simulink model "delay_tuning"  (R2019a)
settings: Solver=VariableStepAuto  StartTime=0.0  StopTime=.05  RelTol=1e-3
values from neighbouring files (symbols this model uses):
  Ari = double(Ari)    [StateSpaceController.m]
  Bri = double(Bri)    [StateSpaceController.m]
  Cri = eye(size(Ari,1))    [StateSpaceController.m]
  Dri = zeros(size(Bri))    [StateSpaceController.m]
  Krv = lqr(Ari, Bri, Qv, diag([0.3 0.3 0.47]) )    [StateSpaceController.m]
  roll_control_delay = ss(Ari, Bri, Cri, Dri, 'InputDelay',[0.07 0.07 0.01])    [StateSpaceController.m]
undefined symbols (not defined in the file or in its folder): e0_0, e1_0, e2_0, e3_0, masscgI
libraries: sharedtransform x3, sharedutil x1
settings Model: Creator=rag  LastModifiedBy=rag

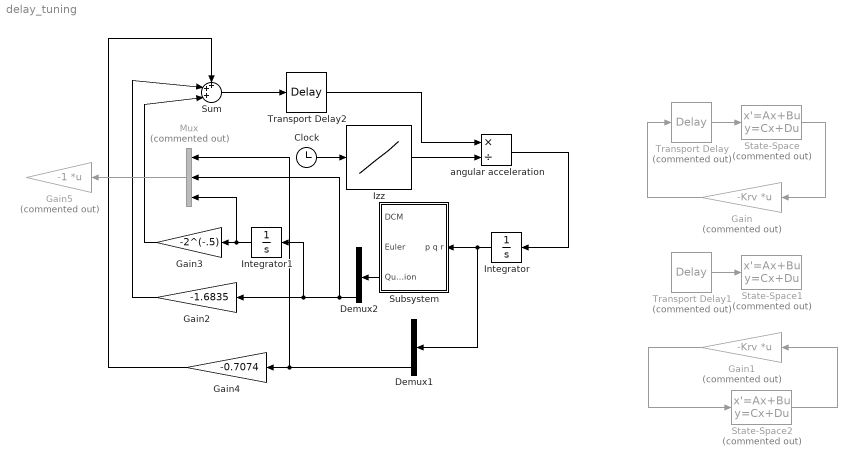
== system delay_tuning ==
  Clock : Clock
  Demux1 : Demux  Outputs=3
  Demux2 : Demux
  Gain : Gain  Commented=on  Gain=-Krv  Multiplication=Matrix(K*u) (u vector)
  Gain1 : Gain  Commented=on  Gain=-Krv  Multiplication=Matrix(K*u) (u vector)
  Gain2 : Gain  Gain=-1.6835
  Gain3 : Gain  Gain=-2^(-.5)
  Gain4 : Gain  Gain=-0.7074
  Gain5 : Gain  Commented=on  Gain=-1  Multiplication=Matrix(K*u) (u vector)
  Integrator : Integrator  InitialCondition=[0; 0; 0.1]
  Integrator1 : Integrator
  Izz : Lookup_n-D  NumberOfTableDimensions=1  BreakpointsForDimension1=masscgI(:,1)  BreakpointsForDimension1FirstPoint=0  BreakpointsForDimension1Spacing=1.5e-5  Table=masscgI(:,4)  InternalRulePriority=Speed  RndMeth=Simplest  InputSameDT=on
  Mux : Mux  Commented=on  Inputs=3
  State-Space : StateSpace  Commented=on  A=Ari  B=Bri  C=Cri  D=Dri  InitialCondition="[.2;.4; -.2;   .2; .1; .3;   .4;.2;.6;   3; -4;  1; -2]"
  State-Space1 : StateSpace  Commented=on  A=Ari  B=Bri  C=Cri  D=Dri  InitialCondition="[.2;.4; -.2;   .2; .1; .3;   .4;.2;.6;   3; -4;  1; -2]"
  State-Space2 : StateSpace  Commented=on  A=roll_control_delay.A  B=roll_control_delay.B  C=roll_control_delay.C  D=roll_control_delay.D  InitialCondition="[.2;.4; -.2;   .2; .1; .3;   .4;.2;.6;   3; -4;  1; -2; 0;0;0]"
  Subsystem : Subsystem
  Sum : Sum  Inputs=+++|
  Transport Delay : TransportDelay  Commented=on  DelayTime=0.07  PadeOrder=5
  Transport Delay1 : TransportDelay  Commented=on  DelayTime=0.07
  Transport Delay2 : TransportDelay  DelayTime=0.07  PadeOrder=5
  angular acceleration : Product  Inputs=*/
  wires:
  State-Space/1 -> Gain/1
  Transport Delay/1 -> State-Space/1
  Gain/1 -> Transport Delay/1
  Gain1/1 -> State-Space2/1
  Transport Delay1/1 -> State-Space1/1
  State-Space2/1 -> Gain1/1
  Clock/1 -> Izz/1
  Izz/1 -> angular acceleration/2
  angular acceleration/1 -> Integrator/1
  Integrator/1 -> Demux1/1, Subsystem/1(p q r)
  Subsystem/3(Quaternion) -> Demux2/1
  Demux2/4 -> Mux/2, Integrator1/1, Gain2/1
  Sum/1 -> Transport Delay2/1
  Gain2/1 -> Sum/2
  Integrator1/1 -> Mux/3, Gain3/1
  Gain3/1 -> Sum/3
  Demux1/3 -> Mux/1, Gain4/1
  Gain4/1 -> Sum/1
  Transport Delay2/1 -> angular acceleration/1
  Mux/1 -> Gain5/1

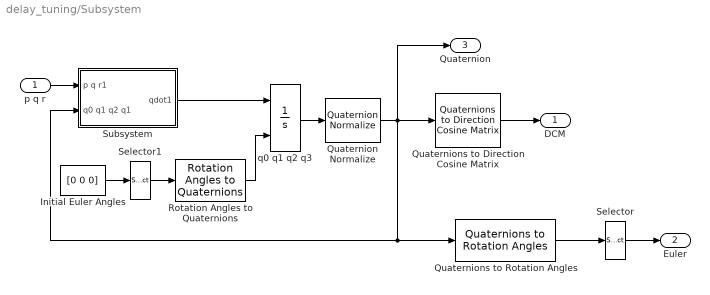
== system delay_tuning/Subsystem ==
  p q r : Inport
  Initial Euler Angles : Constant  Value=[0 0 0]
  Quaternion Normalize : sharedutil/Quaternion Normalize  aMode=aMode
      settings: SourceProductName=Aerospace Blockset  SourceProductBaseCode=AE
  Quaternions to Direction Cosine Matrix : sharedtransform/Quaternions to  Direction Cosine Matrix  aMode=aMode
      settings: SourceProductName=Aerospace Blockset  SourceProductBaseCode=AE
  Quaternions to Rotation Angles : sharedtransform/Quaternions to Rotation Angles  rotationOrder=ZYX  aMode=aMode
      settings: SourceProductBaseCode=AE
  Rotation Angles to Quaternions : sharedtransform/Rotation Angles to Quaternions  rotationOrder=ZYX  aMode=aMode
      settings: SourceProductName=Aerospace Blockset  SourceProductBaseCode=AE
  Selector : Selector  IndexMode=Zero-based  InputPortWidth=3  IndexOptions=Index vector (dialog)  Indices=[ 2 1 0]  OutputSizes=1
  Selector1 : Selector  IndexMode=Zero-based  InputPortWidth=3  IndexOptions=Index vector (dialog)  Indices=[2 1 0]  OutputSizes=1
  Subsystem : Subsystem
  q0 q1 q2 q3 : Integrator  InitialConditionSource=external  InitialCondition=[e0_0 e1_0 e2_0 e3_0]
  DCM : Outport
  Euler : Outport  Port=2
  Quaternion : Outport  Port=3
  wires:
  Rotation Angles to Quaternions/1 -> q0 q1 q2 q3/2
  Selector/1 -> Euler/1
  Initial Euler Angles/1 -> Selector1/1
  Selector1/1 -> Rotation Angles to Quaternions/1
  q0 q1 q2 q3/1 -> Quaternion Normalize/1
  Quaternions to Direction Cosine Matrix/1 -> DCM/1
  Subsystem/1(qdot1) -> q0 q1 q2 q3/1
  p q r/1 -> Subsystem/1(p q r1)
  Quaternions to Rotation Angles/1 -> Selector/1
  Quaternion Normalize/1 -> Quaternion/1, Subsystem/2(q0 q1 q2 q1), Quaternions to Rotation Angles/1, Quaternions to Direction Cosine Matrix/1

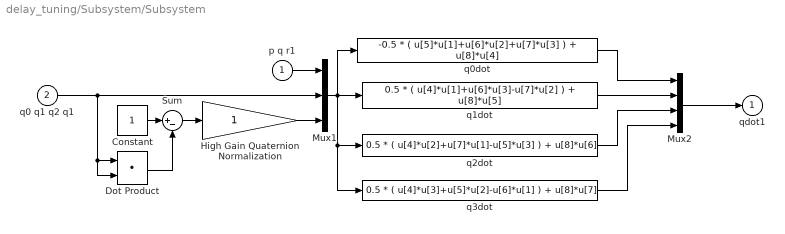
== system delay_tuning/Subsystem/Subsystem ==
  p q r1 : Inport
  q0 q1 q2 q1 : Inport  Port=2
  Constant : Constant
  Dot Product : DotProduct  OutDataTypeStr=Inherit: Inherit via internal rule
  High Gain Quaternion Normalization : Gain  SaturateOnIntegerOverflow=on  OutDataTypeStr=Inherit: Same as input  ParamDataTypeStr=Inherit: Same as input
  Mux1 : Mux  Inputs=[3 4 1]
  Mux2 : Mux
  Sum : Sum  Inputs=|+-  SaturateOnIntegerOverflow=on  InputSameDT=on  OutDataTypeStr=Inherit: Same as first input
  q0dot : Fcn  Expr=-0.5 * ( u[5]*u[1]+u[6]*u[2]+u[7]*u[3] ) + u[8]*u[4]
  q1dot : Fcn  Expr=0.5 * ( u[4]*u[1]+u[6]*u[3]-u[7]*u[2] ) + u[8]*u[5]
  q2dot : Fcn  Expr=0.5 * ( u[4]*u[2]+u[7]*u[1]-u[5]*u[3] ) + u[8]*u[6]
  q3dot : Fcn  Expr=0.5 * ( u[4]*u[3]+u[5]*u[2]-u[6]*u[1] ) + u[8]*u[7]
  qdot1 : Outport  InitialOutput=0
  wires:
  Constant/1 -> Sum/1
  Dot Product/1 -> Sum/2
  Mux1/1 -> q2dot/1, q3dot/1, q0dot/1, q1dot/1
  q0 q1 q2 q1/1 -> Dot Product/1, Dot Product/2, Mux1/2
  Sum/1 -> High Gain Quaternion Normalization/1
  Mux2/1 -> qdot1/1
  q0dot/1 -> Mux2/1
  q3dot/1 -> Mux2/4
  q1dot/1 -> Mux2/2
  q2dot/1 -> Mux2/3
  High Gain Quaternion Normalization/1 -> Mux1/3
  p q r1/1 -> Mux1/1
